simulink model "Topo_03_pcm"  (R2013a)
settings: Solver=ode45  StartTime=0.0  StopTime=10.0  RelTol=1e-6
undefined symbols (not defined in the file): magnitude
(part 2 of 2)

== system Topo_03_pcm/Subsystem1/Subsystem/ACPO_HL/Subsystem/R0 ==
  x : Inport
  y : Inport  Port=2
  theta : Inport  Port=3
  MATLAB Function1 : MATLAB Function  TreatAsAtomicUnit=on
  xr : Outport
  yr : Outport  Port=2
  wires:
  x/1 -> MATLAB Function1/1(x)
  y/1 -> MATLAB Function1/2(y)
  theta/1 -> MATLAB Function1/3(theta)
  MATLAB Function1/1(xr) -> xr/1
  MATLAB Function1/2(yr) -> yr/1

== system Topo_03_pcm/Subsystem1/Subsystem/ACPO_HL/Subsystem/R1 ==
  x : Inport
  y : Inport  Port=2
  theta : Inport  Port=3
  MATLAB Function1 : MATLAB Function  TreatAsAtomicUnit=on
  xr : Outport
  yr : Outport  Port=2
  wires:
  x/1 -> MATLAB Function1/1(x)
  y/1 -> MATLAB Function1/2(y)
  theta/1 -> MATLAB Function1/3(theta)
  MATLAB Function1/1(xr) -> xr/1
  MATLAB Function1/2(yr) -> yr/1

== system Topo_03_pcm/Subsystem1/Subsystem/ACPO_HL/Subsystem/RX ==
  x : Inport
  y : Inport  Port=2
  theta : Inport  Port=3
  MATLAB Function1 : MATLAB Function  TreatAsAtomicUnit=on
  xr : Outport
  yr : Outport  Port=2
  wires:
  x/1 -> MATLAB Function1/1(x)
  y/1 -> MATLAB Function1/2(y)
  theta/1 -> MATLAB Function1/3(theta)
  MATLAB Function1/1(xr) -> xr/1
  MATLAB Function1/2(yr) -> yr/1

== system Topo_03_pcm/Subsystem1/Subsystem/ACPO_HL/Subsystem/RXX ==
  x : Inport
  y : Inport  Port=2
  theta : Inport  Port=3
  MATLAB Function1 : MATLAB Function  TreatAsAtomicUnit=on
  xr : Outport
  yr : Outport  Port=2
  wires:
  x/1 -> MATLAB Function1/1(x)
  y/1 -> MATLAB Function1/2(y)
  theta/1 -> MATLAB Function1/3(theta)
  MATLAB Function1/1(xr) -> xr/1
  MATLAB Function1/2(yr) -> yr/1

== system Topo_03_pcm/Subsystem1/Subsystem/ACPO_HR /Subsystem/R0 ==
  x : Inport
  y : Inport  Port=2
  theta : Inport  Port=3
  MATLAB Function1 : MATLAB Function  TreatAsAtomicUnit=on
  xr : Outport
  yr : Outport  Port=2
  wires:
  x/1 -> MATLAB Function1/1(x)
  y/1 -> MATLAB Function1/2(y)
  theta/1 -> MATLAB Function1/3(theta)
  MATLAB Function1/1(xr) -> xr/1
  MATLAB Function1/2(yr) -> yr/1

== system Topo_03_pcm/Subsystem1/Subsystem/ACPO_HR /Subsystem/R2 ==
  x : Inport
  y : Inport  Port=2
  theta : Inport  Port=3
  MATLAB Function1 : MATLAB Function  TreatAsAtomicUnit=on
  xr : Outport
  yr : Outport  Port=2
  wires:
  x/1 -> MATLAB Function1/1(x)
  y/1 -> MATLAB Function1/2(y)
  theta/1 -> MATLAB Function1/3(theta)
  MATLAB Function1/1(xr) -> xr/1
  MATLAB Function1/2(yr) -> yr/1

== system Topo_03_pcm/Subsystem1/Subsystem/ACPO_HR /Subsystem/RX ==
  x : Inport
  y : Inport  Port=2
  theta : Inport  Port=3
  MATLAB Function1 : MATLAB Function  TreatAsAtomicUnit=on
  xr : Outport
  yr : Outport  Port=2
  wires:
  x/1 -> MATLAB Function1/1(x)
  y/1 -> MATLAB Function1/2(y)
  theta/1 -> MATLAB Function1/3(theta)
  MATLAB Function1/1(xr) -> xr/1
  MATLAB Function1/2(yr) -> yr/1

== system Topo_03_pcm/Subsystem1/Subsystem/ACPO_HR /Subsystem/RXX ==
  x : Inport
  y : Inport  Port=2
  theta : Inport  Port=3
  MATLAB Function1 : MATLAB Function  TreatAsAtomicUnit=on
  xr : Outport
  yr : Outport  Port=2
  wires:
  x/1 -> MATLAB Function1/1(x)
  y/1 -> MATLAB Function1/2(y)
  theta/1 -> MATLAB Function1/3(theta)
  MATLAB Function1/1(xr) -> xr/1
  MATLAB Function1/2(yr) -> yr/1

== system Topo_03_pcm/Subsystem1/Subsystem/ACPO_KL/Subsystem/R0 ==
  x : Inport
  y : Inport  Port=2
  theta : Inport  Port=3
  MATLAB Function1 : MATLAB Function  TreatAsAtomicUnit=on
  xr : Outport
  yr : Outport  Port=2
  wires:
  x/1 -> MATLAB Function1/1(x)
  y/1 -> MATLAB Function1/2(y)
  theta/1 -> MATLAB Function1/3(theta)
  MATLAB Function1/1(xr) -> xr/1
  MATLAB Function1/2(yr) -> yr/1

== system Topo_03_pcm/Subsystem1/Subsystem/ACPO_KL/Subsystem/R4 ==
  x : Inport
  y : Inport  Port=2
  theta : Inport  Port=3
  MATLAB Function1 : MATLAB Function  TreatAsAtomicUnit=on
  xr : Outport
  yr : Outport  Port=2
  wires:
  x/1 -> MATLAB Function1/1(x)
  y/1 -> MATLAB Function1/2(y)
  theta/1 -> MATLAB Function1/3(theta)
  MATLAB Function1/1(xr) -> xr/1
  MATLAB Function1/2(yr) -> yr/1

== system Topo_03_pcm/Subsystem1/Subsystem/ACPO_KL/Subsystem/RX ==
  x : Inport
  y : Inport  Port=2
  theta : Inport  Port=3
  MATLAB Function1 : MATLAB Function  TreatAsAtomicUnit=on
  xr : Outport
  yr : Outport  Port=2
  wires:
  x/1 -> MATLAB Function1/1(x)
  y/1 -> MATLAB Function1/2(y)
  theta/1 -> MATLAB Function1/3(theta)
  MATLAB Function1/1(xr) -> xr/1
  MATLAB Function1/2(yr) -> yr/1

== system Topo_03_pcm/Subsystem1/Subsystem/ACPO_KL/Subsystem/RXX ==
  x : Inport
  y : Inport  Port=2
  theta : Inport  Port=3
  MATLAB Function1 : MATLAB Function  TreatAsAtomicUnit=on
  xr : Outport
  yr : Outport  Port=2
  wires:
  x/1 -> MATLAB Function1/1(x)
  y/1 -> MATLAB Function1/2(y)
  theta/1 -> MATLAB Function1/3(theta)
  MATLAB Function1/1(xr) -> xr/1
  MATLAB Function1/2(yr) -> yr/1

== system Topo_03_pcm/Subsystem1/Subsystem/ACPO_KR/Subsystem/R0 ==
  x : Inport
  y : Inport  Port=2
  theta : Inport  Port=3
  MATLAB Function1 : MATLAB Function  TreatAsAtomicUnit=on
  xr : Outport
  yr : Outport  Port=2
  wires:
  x/1 -> MATLAB Function1/1(x)
  y/1 -> MATLAB Function1/2(y)
  theta/1 -> MATLAB Function1/3(theta)
  MATLAB Function1/1(xr) -> xr/1
  MATLAB Function1/2(yr) -> yr/1

== system Topo_03_pcm/Subsystem1/Subsystem/ACPO_KR/Subsystem/R3 ==
  x : Inport
  y : Inport  Port=2
  theta : Inport  Port=3
  MATLAB Function1 : MATLAB Function  TreatAsAtomicUnit=on
  xr : Outport
  yr : Outport  Port=2
  wires:
  x/1 -> MATLAB Function1/1(x)
  y/1 -> MATLAB Function1/2(y)
  theta/1 -> MATLAB Function1/3(theta)
  MATLAB Function1/1(xr) -> xr/1
  MATLAB Function1/2(yr) -> yr/1

== system Topo_03_pcm/Subsystem1/Subsystem/ACPO_KR/Subsystem/RX ==
  x : Inport
  y : Inport  Port=2
  theta : Inport  Port=3
  MATLAB Function1 : MATLAB Function  TreatAsAtomicUnit=on
  xr : Outport
  yr : Outport  Port=2
  wires:
  x/1 -> MATLAB Function1/1(x)
  y/1 -> MATLAB Function1/2(y)
  theta/1 -> MATLAB Function1/3(theta)
  MATLAB Function1/1(xr) -> xr/1
  MATLAB Function1/2(yr) -> yr/1

== system Topo_03_pcm/Subsystem1/Subsystem/ACPO_KR/Subsystem/RXX ==
  x : Inport
  y : Inport  Port=2
  theta : Inport  Port=3
  MATLAB Function1 : MATLAB Function  TreatAsAtomicUnit=on
  xr : Outport
  yr : Outport  Port=2
  wires:
  x/1 -> MATLAB Function1/1(x)
  y/1 -> MATLAB Function1/2(y)
  theta/1 -> MATLAB Function1/3(theta)
  MATLAB Function1/1(xr) -> xr/1
  MATLAB Function1/2(yr) -> yr/1

== system Topo_03_pcm/Subsystem1/Subsystem/ACPO_RIB/Subsystem/R1 ==
  x : Inport
  y : Inport  Port=2
  theta : Inport  Port=3
  MATLAB Function1 : MATLAB Function  TreatAsAtomicUnit=on
  xr : Outport
  yr : Outport  Port=2
  wires:
  x/1 -> MATLAB Function1/1(x)
  y/1 -> MATLAB Function1/2(y)
  theta/1 -> MATLAB Function1/3(theta)
  MATLAB Function1/1(xr) -> xr/1
  MATLAB Function1/2(yr) -> yr/1

== system Topo_03_pcm/Subsystem1/Subsystem/ACPO_RIB/Subsystem/R2 ==
  x : Inport
  y : Inport  Port=2
  theta : Inport  Port=3
  MATLAB Function1 : MATLAB Function  TreatAsAtomicUnit=on
  xr : Outport
  yr : Outport  Port=2
  wires:
  x/1 -> MATLAB Function1/1(x)
  y/1 -> MATLAB Function1/2(y)
  theta/1 -> MATLAB Function1/3(theta)
  MATLAB Function1/1(xr) -> xr/1
  MATLAB Function1/2(yr) -> yr/1

== matlab function Topo_03_pcm/Subsystem1/Subsystem/ACPO_HL/Subsystem/RX/MATLAB Function1 ==
  data: x input; y input; theta input; xr output; yr output
function [xr,yr]=Rot_theta(x,y,theta)
xr=[cos(theta) -sin(theta)]*[x y]';
yr=[sin(theta) cos(theta)]*[x y]';
end

== matlab function Topo_03_pcm/Subsystem1/MATLAB Function ==
  data: phi input; pcm output
function pcm=pcm(phi)
g=phi.*180./pi;
for i=1:length(g)
    if g(i)<0 
        g(i)=g(i)+360;
    end
end
pcm=g.*100./(360);

== matlab function Topo_03_pcm/Subsystem1/Subsystem/ACPO_HL/Subsystem/RXX/MATLAB Function1 ==
  data: x input; y input; theta input; xr output; yr output
function [xr,yr]=Rot_theta(x,y,theta)
xr=[cos(theta) -sin(theta)]*[x y]';
yr=[sin(theta) cos(theta)]*[x y]';
end

== matlab function Topo_03_pcm/Subsystem1/Subsystem/ACPO_HL/Subsystem/R0/MATLAB Function1 ==
  data: x input; y input; theta input; xr output; yr output
function [xr,yr]=Rot_theta(x,y,theta)
xr=[cos(theta) -sin(theta)]*[x y]';
yr=[sin(theta) cos(theta)]*[x y]';
end

== matlab function Topo_03_pcm/Subsystem1/Subsystem/ACPO_HR /Subsystem/RX/MATLAB Function1 ==
  data: x input; y input; theta input; xr output; yr output
function [xr,yr]=Rot_theta(x,y,theta)
xr=[cos(theta) -sin(theta)]*[x y]';
yr=[sin(theta) cos(theta)]*[x y]';
end

== matlab function Topo_03_pcm/Subsystem1/Subsystem/ACPO_HR /Subsystem/RXX/MATLAB Function1 ==
  data: x input; y input; theta input; xr output; yr output
function [xr,yr]=Rot_theta(x,y,theta)
xr=[cos(theta) -sin(theta)]*[x y]';
yr=[sin(theta) cos(theta)]*[x y]';
end

== matlab function Topo_03_pcm/Subsystem1/Subsystem/ACPO_HR /Subsystem/R0/MATLAB Function1 ==
  data: x input; y input; theta input; xr output; yr output
function [xr,yr]=Rot_theta(x,y,theta)
xr=[cos(theta) -sin(theta)]*[x y]';
yr=[sin(theta) cos(theta)]*[x y]';
end

== matlab function Topo_03_pcm/Subsystem1/Subsystem/ACPO_KR/Subsystem/RXX/MATLAB Function1 ==
  data: x input; y input; theta input; xr output; yr output
function [xr,yr]=Rot_theta(x,y,theta)
xr=[cos(theta) -sin(theta)]*[x y]';
yr=[sin(theta) cos(theta)]*[x y]';
end

== matlab function Topo_03_pcm/Subsystem1/Subsystem/ACPO_KR/Subsystem/RX/MATLAB Function1 ==
  data: x input; y input; theta input; xr output; yr output
function [xr,yr]=Rot_theta(x,y,theta)
xr=[cos(theta) -sin(theta)]*[x y]';
yr=[sin(theta) cos(theta)]*[x y]';
end

== matlab function Topo_03_pcm/Subsystem1/Subsystem/ACPO_KL/Subsystem/R0/MATLAB Function1 ==
  data: x input; y input; theta input; xr output; yr output
function [xr,yr]=Rot_theta(x,y,theta)
xr=[cos(theta) -sin(theta)]*[x y]';
yr=[sin(theta) cos(theta)]*[x y]';
end

== matlab function Topo_03_pcm/Subsystem1/Subsystem/ACPO_KL/Subsystem/RX/MATLAB Function1 ==
  data: x input; y input; theta input; xr output; yr output
function [xr,yr]=Rot_theta(x,y,theta)
xr=[cos(theta) -sin(theta)]*[x y]';
yr=[sin(theta) cos(theta)]*[x y]';
end

== matlab function Topo_03_pcm/Subsystem1/Subsystem/ACPO_KL/Subsystem/RXX/MATLAB Function1 ==
  data: x input; y input; theta input; xr output; yr output
function [xr,yr]=Rot_theta(x,y,theta)
xr=[cos(theta) -sin(theta)]*[x y]';
yr=[sin(theta) cos(theta)]*[x y]';
end

== matlab function Topo_03_pcm/Subsystem1/Subsystem/ACPO_KR/Subsystem/R0/MATLAB Function1 ==
  data: x input; y input; theta input; xr output; yr output
function [xr,yr]=Rot_theta(x,y,theta)
xr=[cos(theta) -sin(theta)]*[x y]';
yr=[sin(theta) cos(theta)]*[x y]';
end

== matlab function Topo_03_pcm/Subsystem1/MATLAB Function1 ==
  data: phi input; pcm output
function pcm=pcm(phi)
g=phi.*180./pi;
for i=1:length(g)
    if g(i)<0 
        g(i)=g(i)+360;
    end
end
pcm=g.*100./(360);

== matlab function Topo_03_pcm/Subsystem1/MATLAB Function2 ==
  data: phi input; pcm output
function pcm=pcm(phi)
g=phi.*180./pi;
for i=1:length(g)
    if g(i)<0 
        g(i)=g(i)+360;
    end
end
pcm=g.*100./(360);

== matlab function Topo_03_pcm/Subsystem1/MATLAB Function3 ==
  data: phi input; pcm output
function pcm=pcm(phi)
g=phi.*180./pi;
for i=1:length(g)
    if g(i)<0 
        g(i)=g(i)+360;
    end
end
pcm=g.*100./(360);

== matlab function Topo_03_pcm/Subsystem1/Subsystem/ACPO_RIB/Subsystem/R2/MATLAB Function1 ==
  data: x input; y input; theta input; xr output; yr output
function [xr,yr]=Rot_theta(x,y,theta)
xr=[cos(theta) -sin(theta)]*[x y]';
yr=[sin(theta) cos(theta)]*[x y]';
end

== matlab function Topo_03_pcm/Subsystem1/Subsystem/ACPO_RIB/Subsystem/R1/MATLAB Function1 ==
  data: x input; y input; theta input; xr output; yr output
function [xr,yr]=Rot_theta(x,y,theta)
xr=[cos(theta) -sin(theta)]*[x y]';
yr=[sin(theta) cos(theta)]*[x y]';
end

== matlab function Topo_03_pcm/Subsystem1/Subsystem/ACPO_HL/Subsystem/R1/MATLAB Function1 ==
  data: x input; y input; theta input; xr output; yr output
function [xr,yr]=Rot_theta(x,y,theta)
xr=[cos(theta) -sin(theta)]*[x y]';
yr=[sin(theta) cos(theta)]*[x y]';
end

== matlab function Topo_03_pcm/Subsystem1/Subsystem/ACPO_HR /Subsystem/R2/MATLAB Function1 ==
  data: x input; y input; theta input; xr output; yr output
function [xr,yr]=Rot_theta(x,y,theta)
xr=[cos(theta) -sin(theta)]*[x y]';
yr=[sin(theta) cos(theta)]*[x y]';
end

== matlab function Topo_03_pcm/Subsystem1/Subsystem/ACPO_KR/Subsystem/R3/MATLAB Function1 ==
  data: x input; y input; theta input; xr output; yr output
function [xr,yr]=Rot_theta(x,y,theta)
xr=[cos(theta) -sin(theta)]*[x y]';
yr=[sin(theta) cos(theta)]*[x y]';
end

== matlab function Topo_03_pcm/Subsystem1/Subsystem/ACPO_KL/Subsystem/R4/MATLAB Function1 ==
  data: x input; y input; theta input; xr output; yr output
function [xr,yr]=Rot_theta(x,y,theta)
xr=[cos(theta) -sin(theta)]*[x y]';
yr=[sin(theta) cos(theta)]*[x y]';
end

== matlab function Topo_03_pcm/Subsystem1/MATLAB Function4 ==
  data: phi input; pcm output
function pcm=pcm(phi)
g=phi.*180./pi;
for i=1:length(g)
    if g(i)<0 
        g(i)=g(i)+360;
    end
end
pcm=g.*100./(360);
